simulink model "Combined_models_Gen_wo_Inertia"  (R2020b)
settings: Solver=VariableStepAuto  StartTime=0.0  StopTime=0.4  EnableMultiTasking=on
undefined symbols (not defined in the file): heaviside, I_const, tau_syn
libraries: NeuroModelerLibrary x8
settings Model: Creator=Bakhshiev  LastModifiedBy=Александра
settings SolverCC: ZeroCrossAlgorithm=Adaptive
settings DataIOCC: LimitDataPoints=on  SaveFormat=Array  SignalLoggingSaveFormat=ModelDataLogs  ReturnWorkspaceOutputs=off
settings OptimizationCC: ExpressionDepthLimit=2147483647  InitFltsAndDblsToZero=on  LifeSpan=inf
settings DebuggingCC: UnderspecifiedInitializationDetection=Classic  MergeDetectMultiDrivingBlocksExec=none  SolverPrmCheckMsg=warning  FcnCallInpInsideContextMsg=warning  StateNameClashWarn=warning  SFUnexpectedBacktrackingDiag=warning  SFNoUnconditionalDefaultTransitionDiag=warning  SFExecutionAtInitializationDiag=none  ArithmeticOperatorsInVariantConditions=warning
settings HardwareCC: ProdBitPerPointer=32  ProdBitPerSizeT=32  ProdBitPerPtrDiffT=32  ProdLargestAtomicFloat=None  ProdIntDivRoundTo=Undefined  ProdEndianess=Unspecified  ProdWordSize=32  ProdHWDeviceType=32-bit Generic
settings ModelReferenceCC: PropagateSignalLabelsOutOfModel=off
settings CodeAppCC: StateflowObjectComments=on
settings GRTTargetCC: TargetLangStandard=C89/C90 (ANSI)  CombineOutputUpdateFcns=off  GRTInterface=on
settings ConfigComp: CovMetricSettings=dw  CovSaveCumulativeToWorkspaceVar=on  CovSaveSingleToWorkspaceVar=on

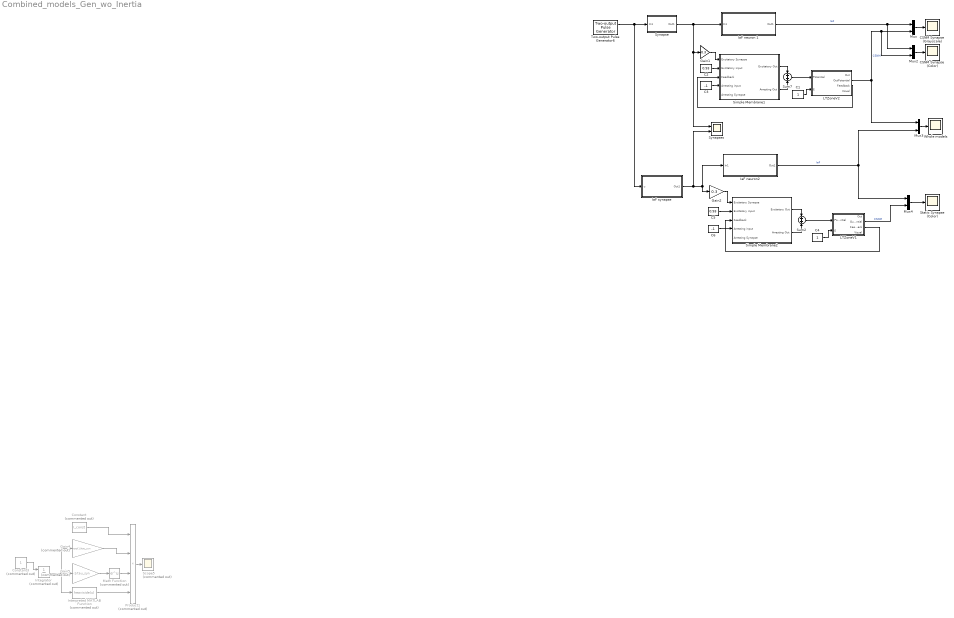
== system Combined_models_Gen_wo_Inertia ==
  C1 : Constant
  C2 : Constant  Value=0.93
  C3 : Constant  Value=-1
  C4 : Constant
  C5 : Constant  Value=0.93
  C6 : Constant  Value=-1
  CSNM Synapse (Color) : Scope
  CSNM Synapse (Grayscale) : Scope
  Constant : Constant  Commented=on  Value=I_const
  Constant3 : Constant  Commented=on
  Gain1 : Gain  Gain=0.3
  Gain2 : Gain  Gain=0.3
  Gain4 : Gain  Commented=on  Gain=exp(1)/tau_syn
  Gain5 : Gain  Commented=on  Gain=-1/tau_syn
  IaF neuron 1 : Subsystem  mask{tau_m=0.01, Cm=250e-12, I_const=0, E_L=-0.070, V_reset=-0.10, V_th=-0.055}
      mask prompts: tau_m "Membrane time constatnt"; Cm "Membrane capacity"; I_const "Constant input current"; E_L "Resting membrane potential"; V_reset "Reset membrane potential"; V_th "Threshold potential"
  IaF neuron2 : Subsystem  mask{tau_m=0.01, Cm=250e-12, I_const=0, E_L=-0.070, V_reset=-0.10, V_th=-0.055}
      mask prompts: tau_m "Membrane time constatnt"; Cm "Membrane capacity"; I_const "Constant input current"; E_L "Resting membrane potential"; V_reset "Reset membrane potential"; V_th "Threshold potential"
  IaF synapse : Subsystem  mask{tau_syn=2e-3, I_syn=1e-8, weight=1, delay=1e-3}
      mask prompts: tau_syn "Rise time of the excitatory synaptic alpha function"; I_syn "Synaptic current amplitude"
  Integrator : Integrator  Commented=on  ExternalReset=falling
  Interpreted MATLAB Function : MATLABFcn  Commented=on  MATLABFcn=heaviside(u)  OutputSignalType=real  Output1D=off
  LTZoneV1 : Subsystem  mask(Ion pump){NM=1, FB=2, T=-0.055, switchOff=-0.1}
      mask prompts: NM "Number of Input Membranes"; FB "Feedback Coeff"; T "On Threshold"; switchOff "Off Threshold"
      mask DialogControl Container3 Prompt: Relay
  LTZoneV2 : Subsystem  mask(Ion pump){NM=1, FB=2, T=-0.055, switchOff=-0.1}
      mask prompts: NM "Number of Input Membranes"; FB "Feedback Coeff"; T "On Threshold"; switchOff "Off Threshold"
      mask DialogControl Container3 Prompt: Relay
  Math Function : Math  Commented=on  SaturateOnIntegerOverflow=on
  Mux : Mux  Inputs=2
  Mux2 : Mux  Inputs=2
  Mux3 : Mux  Inputs=3
  Mux4 : Mux  Inputs=2
  Product1 : Product  Commented=on  Inputs=4
  Scope5 : Scope  Commented=on
  Simple Membrane1 : Subsystem  mask{ACm=1e-9, ARm=1e7, ECm=1e-9, ERm=1e7, ARFm=1e7, ERFm=1e7, U0=-0.070, sign=-1}
      mask prompts: ACm "Arresting Membrane Capacity"; ARm "Arresting Membrane Resistance"; ECm "Excitatory Membrane Capacity"; ERm "Excitatory Membrane Resistance"; ARFm "Feedback Arresting Resistance"; ERFm "Feedback Excitatory Resistance"; U0 "Synaptic potential"; sign "Synaptic current sign"
  Simple Membrane2 : Subsystem  mask{ACm=1e-9, ARm=1e7, ECm=1e-9, ERm=1e7, ARFm=1e7, ERFm=1e7, U0=-0.070, sign=-1}
      mask prompts: ACm "Arresting Membrane Capacity"; ARm "Arresting Membrane Resistance"; ECm "Excitatory Membrane Capacity"; ERm "Excitatory Membrane Resistance"; ARFm "Feedback Arresting Resistance"; ERFm "Feedback Excitatory Resistance"; U0 "Synaptic potential"; sign "Synaptic current sign"
  Static Synapse (Color) : Scope
  Sum2 : Sum  InputSameDT=on  SaturateOnIntegerOverflow=on  OutDataTypeStr=Inherit: Same as first input
  Sum7 : Sum  InputSameDT=on  SaturateOnIntegerOverflow=on  OutDataTypeStr=Inherit: Same as first input
  Synapse : Subsystem  mask{SecretionTC=0.001, DecompositionTC=0.005, UseKsi=off, gamma=2e7, ksi=1, U0=-0.070, weight=1, sign=off}
      mask prompts: SecretionTC "Mediator Secretion"; DecompositionTC "Mediator Decomposition"; UseKsi "Use Presynaptic Inhubition"; U0 "Synaptic potential"; weight "Synaptic weight"; sign "Negative synaptic current"
  Synapses : Scope  NumInputPorts=2
  Two-output Pulse Generator6 : NeuroModelerLibrary/Support/Two-output Pulse Generator  A=1  P1=200  P2=200  PW=1  ST=0.001  OOn1=0.1  OOff1=1.0  OOn2=0.1  OOff2=0.2
  Whole models : Scope
  wires:
  Simple Membrane1/1(Excitatory Out) -> Sum7/1
  Simple Membrane1/2(Arresting Out) -> Sum7/2
  LTZoneV2/3(Feedback) -> Simple Membrane1/3(Feedback)
  C1/1 -> LTZoneV2/2(E)
  Sum7/1 -> LTZoneV2/1(Potential)
  Synapse/1(Out1) -> IaF neuron 1/1(In1), Synapses/1, Gain1/1
  Two-output Pulse Generator6/1 -> IaF synapse/1(u), Synapse/1(In1)
  Gain5/1 -> Math Function/1
  Constant/1 -> Product1/1
  Gain4/1 -> Product1/2
  Math Function/1 -> Product1/3
  Product1/1 -> Scope5/1
  Interpreted MATLAB Function/1 -> Product1/4
  Constant3/1 -> Integrator/1
  Integrator/1 -> Interpreted MATLAB Function/1, Gain5/1, Gain4/1
  Simple Membrane2/2(Arresting Out) -> Sum2/2
  C4/1 -> LTZoneV1/2(E)
  Simple Membrane2/1(Excitatory Out) -> Sum2/1
  LTZoneV1/3(Feedback) -> Simple Membrane2/3(Feedback)
  IaF neuron2/1(Out1) -> Mux4/1, Mux3/3  "IaF"
  C5/1 -> Simple Membrane2/2(Excitatory input)
  C6/1 -> Simple Membrane2/4(Arresting input)
  IaF synapse/1(Out1) -> Synapses/2, Gain2/1, IaF neuron2/1(In1)
  Sum2/1 -> LTZoneV1/1(Potential)
  C3/1 -> Simple Membrane1/4(Arresting input)
  C2/1 -> Simple Membrane1/2(Excitatory input)
  IaF neuron 1/1(Out1) -> Mux2/1, Mux/1  "IaF"
  Gain1/1 -> Simple Membrane1/1(Excitatory Synapse)
  Mux/1 -> CSNM Synapse (Grayscale)/1
  LTZoneV2/2(OutPotential) -> Mux3/1, Mux2/2, Mux/2  "CSNM"
  Gain2/1 -> Simple Membrane2/1(Excitatory Synapse)
  LTZoneV1/2(OutPotential) -> Mux4/2  "CSNM"
  Mux3/1 -> Whole models/1
  Mux2/1 -> CSNM Synapse (Color)/1
  Mux4/1 -> Static Synapse (Color)/1

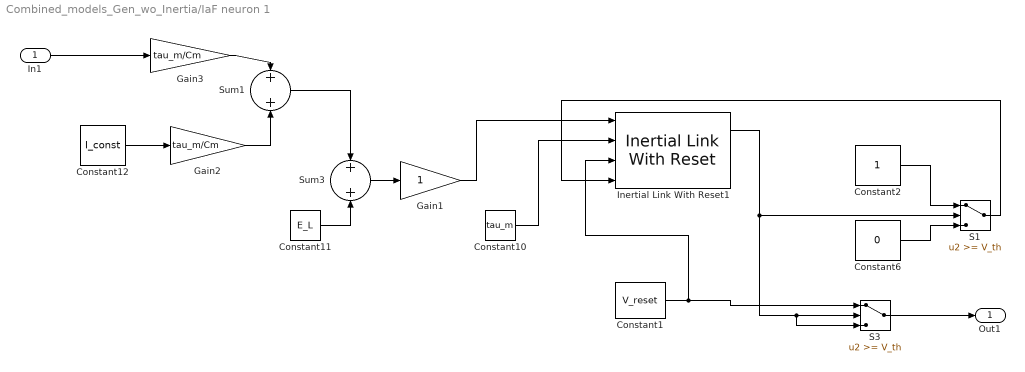
== system Combined_models_Gen_wo_Inertia/IaF neuron 1 ==
  In1 : Inport
  Constant1 : Constant  Value=V_reset
  Constant10 : Constant  Value=tau_m
  Constant11 : Constant  Value=E_L
  Constant12 : Constant  Value=I_const
  Constant2 : Constant
  Constant6 : Constant  Value=0
  Gain1 : Gain
  Gain2 : Gain  Gain=tau_m/Cm
  Gain3 : Gain  Gain=tau_m/Cm
  Inertial Link With Reset1 : NeuroModelerLibrary/Support/Inertial Link With Reset  SystemSampleTime=-1  VariantActivationTime=update diagram  Latency=0  AutoFrameSizeCalculation=off
  S1 : Switch  Threshold=V_th  SaturateOnIntegerOverflow=on  InputSameDT=on
  S3 : Switch  Threshold=V_th  SaturateOnIntegerOverflow=on  InputSameDT=on
  Sum1 : Sum
  Sum3 : Sum
  Out1 : Outport
  wires:
  Constant12/1 -> Gain2/1
  Constant11/1 -> Sum3/2
  Constant10/1 -> Inertial Link With Reset1/2
  Gain3/1 -> Sum1/1
  Sum1/1 -> Sum3/1
  Gain2/1 -> Sum1/2
  Constant2/1 -> S1/1
  Constant6/1 -> S1/3
  Sum3/1 -> Gain1/1
  Gain1/1 -> Inertial Link With Reset1/1
  Inertial Link With Reset1/1 -> S1/2, S3/3, S3/2
  Constant1/1 -> Inertial Link With Reset1/3, S3/1
  S1/1 -> Inertial Link With Reset1/4
  In1/1 -> Gain3/1
  S3/1 -> Out1/1

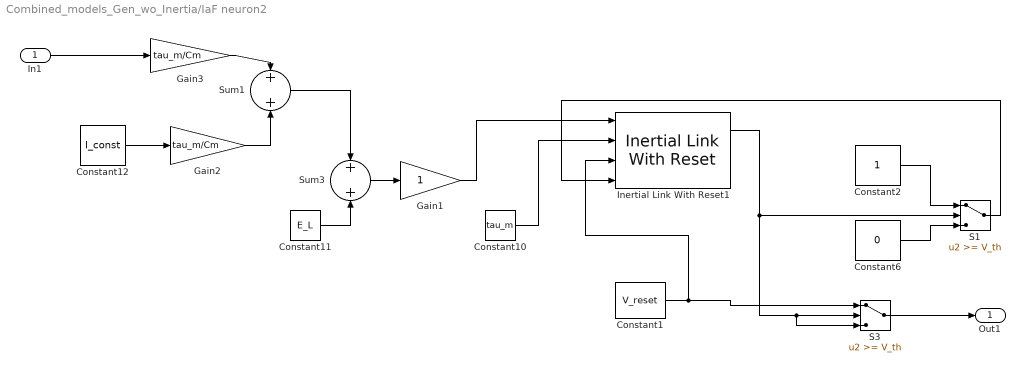
== system Combined_models_Gen_wo_Inertia/IaF neuron2 ==
  In1 : Inport
  Constant1 : Constant  Value=V_reset
  Constant10 : Constant  Value=tau_m
  Constant11 : Constant  Value=E_L
  Constant12 : Constant  Value=I_const
  Constant2 : Constant
  Constant6 : Constant  Value=0
  Gain1 : Gain
  Gain2 : Gain  Gain=tau_m/Cm
  Gain3 : Gain  Gain=tau_m/Cm
  Inertial Link With Reset1 : NeuroModelerLibrary/Support/Inertial Link With Reset  SystemSampleTime=-1  VariantActivationTime=update diagram  Latency=0  AutoFrameSizeCalculation=off
  S1 : Switch  Threshold=V_th  SaturateOnIntegerOverflow=on  InputSameDT=on
  S3 : Switch  Threshold=V_th  SaturateOnIntegerOverflow=on  InputSameDT=on
  Sum1 : Sum
  Sum3 : Sum
  Out1 : Outport
  wires:
  Constant12/1 -> Gain2/1
  Constant11/1 -> Sum3/2
  Constant10/1 -> Inertial Link With Reset1/2
  Gain3/1 -> Sum1/1
  Sum1/1 -> Sum3/1
  Gain2/1 -> Sum1/2
  Constant2/1 -> S1/1
  Constant6/1 -> S1/3
  Sum3/1 -> Gain1/1
  Gain1/1 -> Inertial Link With Reset1/1
  Inertial Link With Reset1/1 -> S1/2, S3/3, S3/2
  Constant1/1 -> Inertial Link With Reset1/3, S3/1
  S1/1 -> Inertial Link With Reset1/4
  In1/1 -> Gain3/1
  S3/1 -> Out1/1

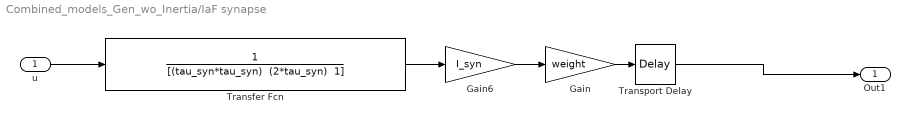
== system Combined_models_Gen_wo_Inertia/IaF synapse ==
  u : Inport
  Gain : Gain  Gain=weight
  Gain6 : Gain  Gain=I_syn
  Transfer Fcn : TransferFcn  Denominator="[(tau_syn*tau_syn)  (2*tau_syn)  1]"
  Transport Delay : TransportDelay  DelayTime=delay
  Out1 : Outport
  wires:
  Transport Delay/1 -> Out1/1
  Gain/1 -> Transport Delay/1
  Gain6/1 -> Gain/1
  Transfer Fcn/1 -> Gain6/1
  u/1 -> Transfer Fcn/1

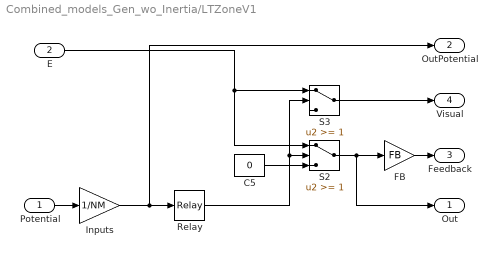
== system Combined_models_Gen_wo_Inertia/LTZoneV1 ==
  Potential : Inport
  E : Inport  Port=2
  C5 : Constant  Value=0
  FB : Gain  Gain=FB  OutDataTypeStr=Inherit: Same as input  ParamDataTypeStr=Inherit: Same as input
  Inputs : Gain  Gain=1/NM  OutDataTypeStr=Inherit: Same as input  ParamDataTypeStr=Inherit: Same as input
  Relay : Relay  OnSwitchValue=T  OffSwitchValue=switchOff
  S2 : Switch  Threshold=1  SaturateOnIntegerOverflow=on  InputSameDT=on
  S3 : Switch  Threshold=1  SaturateOnIntegerOverflow=on  InputSameDT=on
  Out : Outport  InitialOutput=0  VectorParamsAs1DForOutWhenUnconnected=off
  OutPotential : Outport  Port=2  InitialOutput=0  VectorParamsAs1DForOutWhenUnconnected=off
  Feedback : Outport  Port=3  InitialOutput=0  VectorParamsAs1DForOutWhenUnconnected=off
  Visual : Outport  Port=4  InitialOutput=0  VectorParamsAs1DForOutWhenUnconnected=off
  wires:
  FB/1 -> Feedback/1
  Potential/1 -> Inputs/1
  C5/1 -> S2/3
  E/1 -> S3/1, S2/1
  S2/1 -> Out/1, FB/1
  Relay/1 -> S2/2, S3/2
  S3/1 -> Visual/1
  Inputs/1 -> OutPotential/1, Relay/1

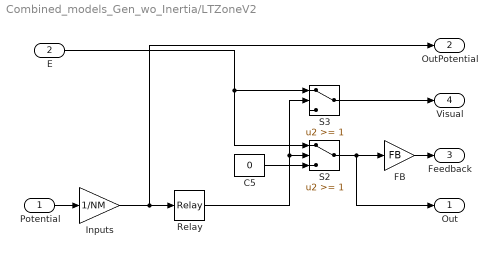
== system Combined_models_Gen_wo_Inertia/LTZoneV2 ==
  Potential : Inport
  E : Inport  Port=2
  C5 : Constant  Value=0
  FB : Gain  Gain=FB  OutDataTypeStr=Inherit: Same as input  ParamDataTypeStr=Inherit: Same as input
  Inputs : Gain  Gain=1/NM  OutDataTypeStr=Inherit: Same as input  ParamDataTypeStr=Inherit: Same as input
  Relay : Relay  OnSwitchValue=T  OffSwitchValue=switchOff
  S2 : Switch  Threshold=1  SaturateOnIntegerOverflow=on  InputSameDT=on
  S3 : Switch  Threshold=1  SaturateOnIntegerOverflow=on  InputSameDT=on
  Out : Outport  InitialOutput=0  VectorParamsAs1DForOutWhenUnconnected=off
  OutPotential : Outport  Port=2  InitialOutput=0  VectorParamsAs1DForOutWhenUnconnected=off
  Feedback : Outport  Port=3  InitialOutput=0  VectorParamsAs1DForOutWhenUnconnected=off
  Visual : Outport  Port=4  InitialOutput=0  VectorParamsAs1DForOutWhenUnconnected=off
  wires:
  FB/1 -> Feedback/1
  Potential/1 -> Inputs/1
  C5/1 -> S2/3
  E/1 -> S3/1, S2/1
  S2/1 -> Out/1, FB/1
  Relay/1 -> S2/2, S3/2
  S3/1 -> Visual/1
  Inputs/1 -> OutPotential/1, Relay/1

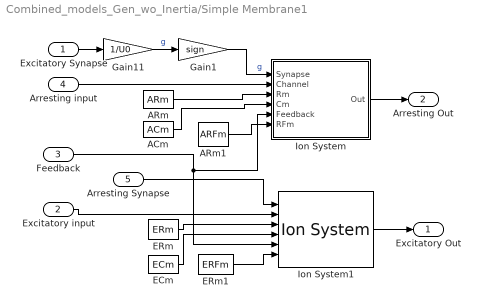
== system Combined_models_Gen_wo_Inertia/Simple Membrane1 ==
  Excitatory Synapse : Inport
  Excitatory input : Inport  Port=2
  Feedback : Inport  Port=3
  Arresting input : Inport  Port=4
  Arresting Synapse : Inport  Port=5
  ACm : Constant  Value=ACm
  ARm : Constant  Value=ARm
  ARm1 : Constant  Value=ARFm
  ECm : Constant  Value=ECm
  ERm : Constant  Value=ERm
  ERm1 : Constant  Value=ERFm
  Gain1 : Gain  Gain=sign
  Gain11 : Gain  Gain=1/U0
  Ion System : Subsystem  AncestorBlock=NeuroModelerLibrary/Neuron Elements/Ion System
  Ion System1 : NeuroModelerLibrary/Neuron Elements/Ion System  SystemSampleTime=-1  VariantActivationTime=update diagram  Latency=0  AutoFrameSizeCalculation=off
  Excitatory Out : Outport  VectorParamsAs1DForOutWhenUnconnected=off
  Arresting Out : Outport  Port=2  VectorParamsAs1DForOutWhenUnconnected=off
  wires:
  Ion System1/1 -> Excitatory Out/1
  ERm1/1 -> Ion System1/6
  Ion System/1(Out) -> Arresting Out/1
  ACm/1 -> Ion System/4(Cm)
  ARm/1 -> Ion System/3(Rm)
  ECm/1 -> Ion System1/4
  ERm/1 -> Ion System1/3
  Excitatory Synapse/1 -> Gain11/1
  Arresting Synapse/1 -> Ion System1/1
  Excitatory input/1 -> Ion System1/2
  ARm1/1 -> Ion System/6(RFm)
  Feedback/1 -> Ion System1/5, Ion System/5(Feedback)
  Arresting input/1 -> Ion System/2(Channel)
  Gain11/1 -> Gain1/1  "g"
  Gain1/1 -> Ion System/1(Synapse)  "g"

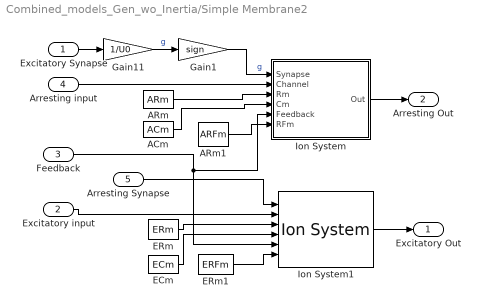
== system Combined_models_Gen_wo_Inertia/Simple Membrane2 ==
  Excitatory Synapse : Inport
  Excitatory input : Inport  Port=2
  Feedback : Inport  Port=3
  Arresting input : Inport  Port=4
  Arresting Synapse : Inport  Port=5
  ACm : Constant  Value=ACm
  ARm : Constant  Value=ARm
  ARm1 : Constant  Value=ARFm
  ECm : Constant  Value=ECm
  ERm : Constant  Value=ERm
  ERm1 : Constant  Value=ERFm
  Gain1 : Gain  Gain=sign
  Gain11 : Gain  Gain=1/U0
  Ion System : Subsystem  AncestorBlock=NeuroModelerLibrary/Neuron Elements/Ion System
  Ion System1 : NeuroModelerLibrary/Neuron Elements/Ion System  SystemSampleTime=-1  VariantActivationTime=update diagram  Latency=0  AutoFrameSizeCalculation=off
  Excitatory Out : Outport  VectorParamsAs1DForOutWhenUnconnected=off
  Arresting Out : Outport  Port=2  VectorParamsAs1DForOutWhenUnconnected=off
  wires:
  Ion System1/1 -> Excitatory Out/1
  ERm1/1 -> Ion System1/6
  Ion System/1(Out) -> Arresting Out/1
  ACm/1 -> Ion System/4(Cm)
  ARm/1 -> Ion System/3(Rm)
  ECm/1 -> Ion System1/4
  ERm/1 -> Ion System1/3
  Excitatory Synapse/1 -> Gain11/1
  Arresting Synapse/1 -> Ion System1/1
  Excitatory input/1 -> Ion System1/2
  ARm1/1 -> Ion System/6(RFm)
  Feedback/1 -> Ion System1/5, Ion System/5(Feedback)
  Arresting input/1 -> Ion System/2(Channel)
  Gain11/1 -> Gain1/1  "g"
  Gain1/1 -> Ion System/1(Synapse)  "g"

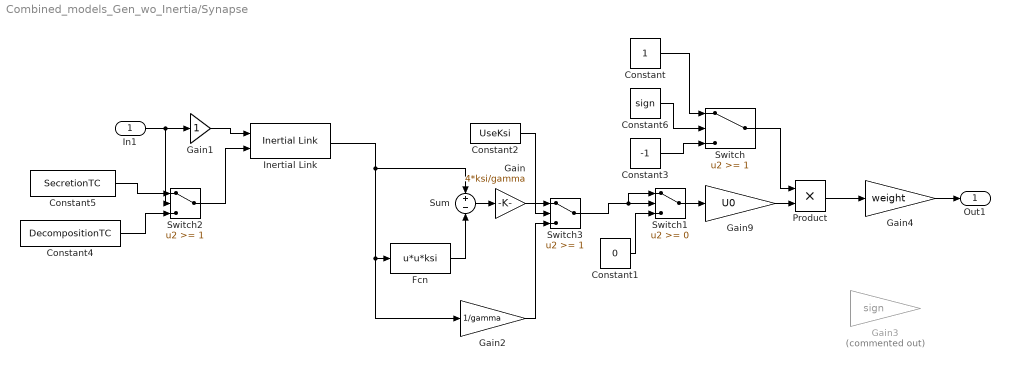
== system Combined_models_Gen_wo_Inertia/Synapse ==
  In1 : Inport
  Constant : Constant
  Constant1 : Constant  Value=0
  Constant2 : Constant  Value=UseKsi
  Constant3 : Constant  Value=-1
  Constant4 : Constant  Value=DecompositionTC
  Constant5 : Constant  Value=SecretionTC
  Constant6 : Constant  Value=sign
  Fcn : Fcn  Expr=u*u*ksi
  Gain : Gain  Gain=4*ksi/gamma  SaturateOnIntegerOverflow=on  OutDataTypeStr=Inherit: Same as input  ParamDataTypeStr=Inherit: Same as input
  Gain1 : Gain  SaturateOnIntegerOverflow=on  OutDataTypeStr=Inherit: Same as input  ParamDataTypeStr=Inherit: Same as input
  Gain2 : Gain  Gain=1/gamma  SaturateOnIntegerOverflow=on  OutDataTypeStr=Inherit: Same as input  ParamDataTypeStr=Inherit: Same as input
  Gain3 : Gain  Commented=on  Gain=sign
  Gain4 : Gain  Gain=weight
  Gain9 : Gain  Gain=U0
  Inertial Link : NeuroModelerLibrary/Support/Inertial Link  SystemSampleTime=-1  VariantActivationTime=update diagram  Latency=0  AutoFrameSizeCalculation=off
  Product : Product
  Sum : Sum  Inputs=+-  SaturateOnIntegerOverflow=on
  Switch : Switch  Threshold=1
  Switch1 : Switch
  Switch2 : Switch  Threshold=1
  Switch3 : Switch  Threshold=1
  Out1 : Outport  VectorParamsAs1DForOutWhenUnconnected=off
  wires:
  Gain2/1 -> Switch3/3
  Constant2/1 -> Switch3/2
  Switch3/1 -> Switch1/2, Switch1/1
  Gain/1 -> Switch3/1
  Switch1/1 -> Gain9/1
  Gain1/1 -> Inertial Link/1
  Constant1/1 -> Switch1/3
  Switch2/1 -> Inertial Link/2
  Constant5/1 -> Switch2/1
  Constant4/1 -> Switch2/3
  Inertial Link/1 -> Sum/1, Fcn/1, Gain2/1
  Sum/1 -> Gain/1
  In1/1 -> Gain1/1, Switch2/2
  Fcn/1 -> Sum/2
  Gain9/1 -> Product/2
  Product/1 -> Gain4/1
  Gain4/1 -> Out1/1
  Switch/1 -> Product/1
  Constant6/1 -> Switch/2
  Constant/1 -> Switch/1
  Constant3/1 -> Switch/3

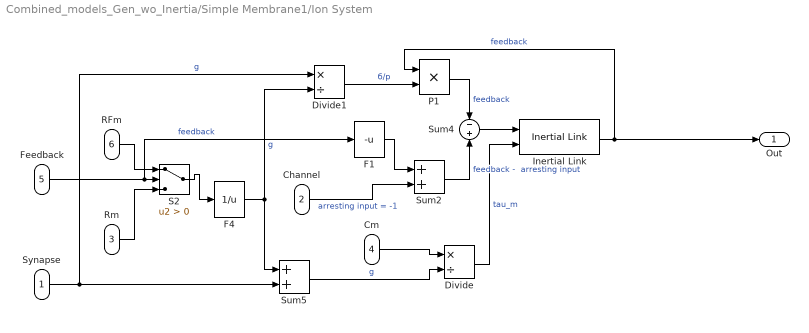
== system Combined_models_Gen_wo_Inertia/Simple Membrane1/Ion System ==
  Synapse : Inport
  Channel : Inport  Port=2
  Rm : Inport  Port=3
  Cm : Inport  Port=4
  Feedback : Inport  Port=5
  RFm : Inport  Port=6
  Divide : Product  Inputs=*/
  Divide1 : Product  Inputs=*/
  F1 : Fcn  Expr=-u
  F4 : Fcn  Expr=1/u
  Inertial Link : NeuroModelerLibrary/Support/Inertial Link  SystemSampleTime=-1  VariantActivationTime=update diagram  Latency=0  AutoFrameSizeCalculation=off
  P1 : Product  InputSameDT=on  RndMeth=Zero  SaturateOnIntegerOverflow=on  OutDataTypeStr=Inherit: Same as first input
  S2 : Switch  Criteria=u2 > Threshold  SaturateOnIntegerOverflow=on  InputSameDT=on
  Sum2 : Sum  InputSameDT=on  SaturateOnIntegerOverflow=on  OutDataTypeStr=Inherit: Same as first input
  Sum4 : Sum  Inputs=-+  InputSameDT=on  SaturateOnIntegerOverflow=on  OutDataTypeStr=Inherit: Same as first input
  Sum5 : Sum  InputSameDT=on  SaturateOnIntegerOverflow=on  OutDataTypeStr=Inherit: Same as first input
  Out : Outport  VectorParamsAs1DForOutWhenUnconnected=off
  wires:
  Divide1/1 -> P1/2  "б/р"
  Cm/1 -> Divide/1
  F4/1 -> Sum5/1, Divide1/2  "g"
  Synapse/1 -> Sum5/2, Divide1/1  "g"
  Divide/1 -> Inertial Link/2  "tau_m"
  Sum5/1 -> Divide/2  "g"
  Inertial Link/1 -> P1/1, Out/1  "feedback"
  P1/1 -> Sum4/1  "feedback"
  Sum4/1 -> Inertial Link/1
  S2/1 -> F4/1
  RFm/1 -> S2/1
  Rm/1 -> S2/3
  Feedback/1 -> S2/2, F1/1  "feedback"
  Sum2/1 -> Sum4/2  "feedback -  arresting input"
  Channel/1 -> Sum2/2  "arresting input = -1"
  F1/1 -> Sum2/1

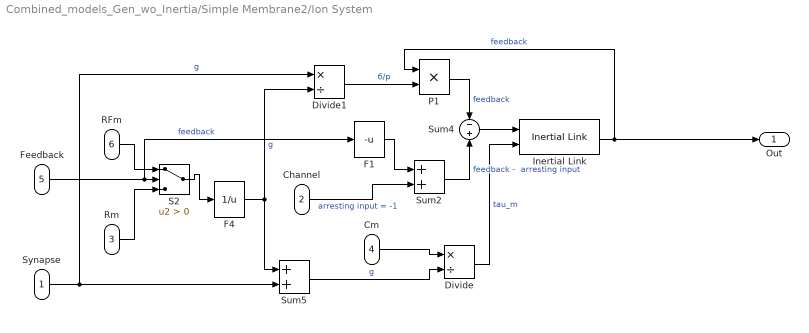
== system Combined_models_Gen_wo_Inertia/Simple Membrane2/Ion System ==
  Synapse : Inport
  Channel : Inport  Port=2
  Rm : Inport  Port=3
  Cm : Inport  Port=4
  Feedback : Inport  Port=5
  RFm : Inport  Port=6
  Divide : Product  Inputs=*/
  Divide1 : Product  Inputs=*/
  F1 : Fcn  Expr=-u
  F4 : Fcn  Expr=1/u
  Inertial Link : NeuroModelerLibrary/Support/Inertial Link  SystemSampleTime=-1  VariantActivationTime=update diagram  Latency=0  AutoFrameSizeCalculation=off
  P1 : Product  InputSameDT=on  RndMeth=Zero  SaturateOnIntegerOverflow=on  OutDataTypeStr=Inherit: Same as first input
  S2 : Switch  Criteria=u2 > Threshold  SaturateOnIntegerOverflow=on  InputSameDT=on
  Sum2 : Sum  InputSameDT=on  SaturateOnIntegerOverflow=on  OutDataTypeStr=Inherit: Same as first input
  Sum4 : Sum  Inputs=-+  InputSameDT=on  SaturateOnIntegerOverflow=on  OutDataTypeStr=Inherit: Same as first input
  Sum5 : Sum  InputSameDT=on  SaturateOnIntegerOverflow=on  OutDataTypeStr=Inherit: Same as first input
  Out : Outport  VectorParamsAs1DForOutWhenUnconnected=off
  wires:
  Divide1/1 -> P1/2  "б/р"
  Cm/1 -> Divide/1
  F4/1 -> Sum5/1, Divide1/2  "g"
  Synapse/1 -> Sum5/2, Divide1/1  "g"
  Divide/1 -> Inertial Link/2  "tau_m"
  Sum5/1 -> Divide/2  "g"
  Inertial Link/1 -> P1/1, Out/1  "feedback"
  P1/1 -> Sum4/1  "feedback"
  Sum4/1 -> Inertial Link/1
  S2/1 -> F4/1
  RFm/1 -> S2/1
  Rm/1 -> S2/3
  Feedback/1 -> S2/2, F1/1  "feedback"
  Sum2/1 -> Sum4/2  "feedback -  arresting input"
  Channel/1 -> Sum2/2  "arresting input = -1"
  F1/1 -> Sum2/1
